simulink model "Radar_Acc_ExtSen_CS9_id"  (Simulink 8.5)
settings: Solver=ode45  StartTime=0  StopTime=50  RelTol=1e-3
libraries: Solver_SF x2, simulink x1
settings Model: Creator=dhall  LastModifiedBy=Mastereal  ExtModeTrigMode=oneshot  ExtModeArmWhenConnect=off
settings DataIOCC: LimitDataPoints=off  SignalLoggingName=sigsOut
settings OptimizationCC: BooleanDataType=off  ExpressionDepthLimit=128  LocalBlockOutputs=off  InitFltsAndDblsToZero=on
settings DebuggingCC: SaveWithParameterizedLinksMsg=none  SignalResolutionControl=TryResolveAllWithWarning  MultiTaskDSMMsg=warning  MultiTaskCondExecSysMsg=none  FcnCallInpInsideContextMsg=UseLocalSettings
settings HardwareCC: TargetUnknown=on
settings GRTTargetCC: TargetFcnLib=ansi_tfl_tmw.mat  CompOptLevelCompliant=off

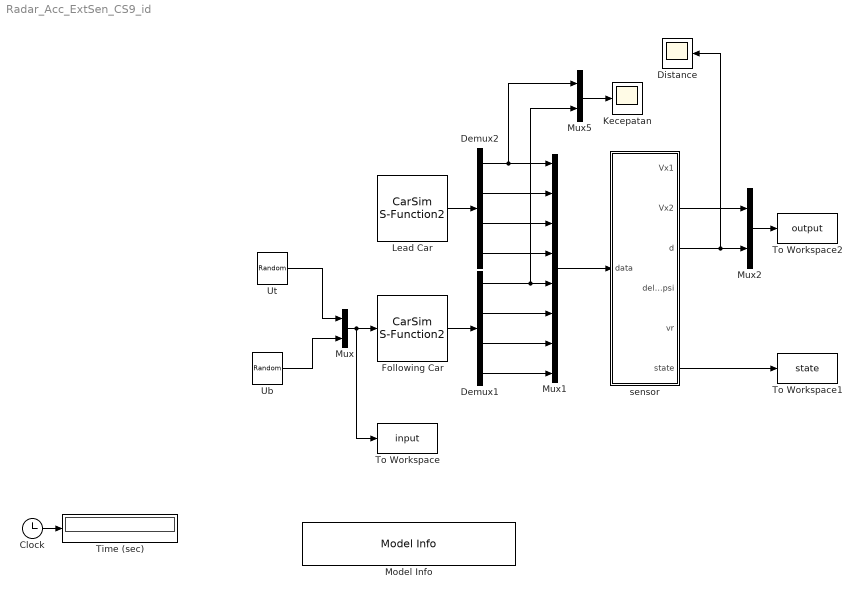
== system Radar_Acc_ExtSen_CS9_id ==
  Clock : Clock
  Demux1 : Demux
  Demux2 : Demux
  Distance : Scope
      settings: TickLabels=on  TimeRange=30  YMin=30  YMax=77.5  SampleTime=100
  Following Car : Solver_SF/CarSim S-Function2  Priority=1  VehicleCode=i_i2  SIMFILE=Radar_Acc_ExtSen_Car_2.sim
      settings: AttributesFormatString=Vehicle Code: %<VehicleCode>
  Kecepatan : Scope
      settings: TickLabels=on  TimeRange=30  YMin=52  YMax=60.5  MaxDataPoints=50000  SampleTime=100
  Lead Car : Solver_SF/CarSim S-Function2  Priority=1  VehicleCode=i_i  SIMFILE=Radar_Acc_ExtSen_Car_1.sim
      settings: AttributesFormatString=Vehicle Code: %<VehicleCode>
  Model Info : simulink/Model-Wide Utilities/Model Info  Frame=on  DisplayStringWithTags=Multi Vehicle Run Adaptive Cruise Control Model  HorizontalTextAlignment=Center  LeftAlignmentValue=0.5  SourceBlockDiagram=Radar_Acc_ExtSen_CS9_id  TagMaxNumber=20
  Mux : Mux  Inputs=2
  Mux1 : Mux  Inputs=8
  Mux2 : Mux  Inputs=2
  Mux5 : Mux  Inputs=2
  Time (sec) : Display
      settings: Format=bank  Decimation=100
  To Workspace : ToWorkspace  VariableName=input  SampleTime=-1
  To Workspace1 : ToWorkspace  VariableName=state  SampleTime=0.002
  To Workspace2 : ToWorkspace  VariableName=output  SampleTime=0.002
  Ub : UniformRandomNumber  Minimum=1.18275  Maximum=1.18775  Seed=200  SampleTime=0.002
  Ut : UniformRandomNumber  Minimum=0.17883  Maximum=0.17887  Seed=200  SampleTime=0.002
  sensor : MATLAB Function  TreatAsAtomicUnit=on
  wires:
  Clock/1 -> Time (sec)/1
  Following Car/1 -> Demux1/1
  Lead Car/1 -> Demux2/1
  Demux2/1 -> Mux1/1, Mux5/1
  Demux2/2 -> Mux1/2
  Demux2/3 -> Mux1/3
  Demux2/4 -> Mux1/4
  Demux1/1 -> Mux5/2, Mux1/5
  Demux1/2 -> Mux1/6
  Demux1/3 -> Mux1/7
  Demux1/4 -> Mux1/8
  Mux1/1 -> sensor/1(data)
  Mux5/1 -> Kecepatan/1
  sensor/2(Vx2) -> Mux2/1
  sensor/3(d) -> Distance/1, Mux2/2
  Mux2/1 -> To Workspace2/1
  sensor/6(state) -> To Workspace1/1
  Ut/1 -> Mux/1
  Ub/1 -> Mux/2
  Mux/1 -> To Workspace/1, Following Car/1

== matlab function sensor ==
  data: data input double; Vx1 output double; Vx2 output double; d output double; delta_psi output double; vr output double; state output double
function [Vx1,Vx2,d,delta_psi,vr,state] = fcn(data)
%#codegen
%pembagian sinyal
Vx1= data(1);
X1= data(2);
Y1= data(3);
psi1= data(4);
Vx2= data(5);
X2= data(6);
Y2= data(7);
psi2= data(8);

psi2fix = mod(psi2,360);

Xo = X1-X2;
Yo = Y1-Y2;
d = sqrt(Xo^2 + Yo^2);
anglerad = atan(Yo/Xo);
anglesudut = anglerad*(180/pi);
sudut = abs(anglesudut-psi2fix);

suduta = sudut;
sudutb = 360 - sudut;

if sudutb >= 270
   delta_psi = suduta;
else 
    delta_psi = sudutb;
end

vr = Vx2-Vx1;

state = [Vx2;d;delta_psi;vr];
